simulink model "bcd_test"  (R2026a)
settings: Solver=ode15s
libraries: scuba_lib x3, nesl_utility x2, fl_lib x1
settings Model: DataDictionary=scubaParams.sldd  Creator=grouleau  LastModifiedBy=grouleau

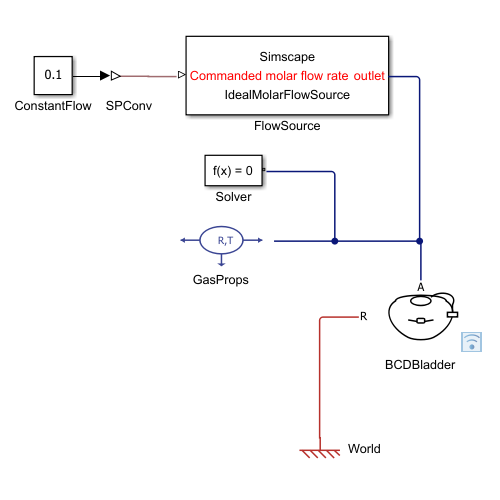
[thumbnail: Simulink's stored preview of the top-level diagram]
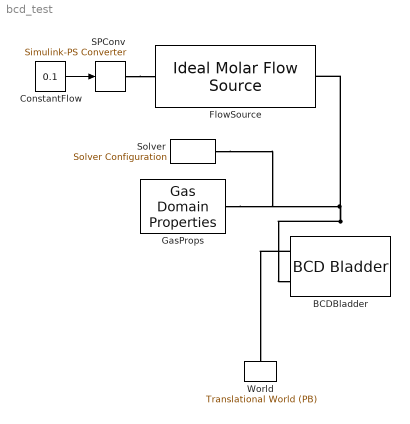
== system bcd_test ==
  BCDBladder : scuba_lib/gas/elements/BCD Bladder  V_max=0.015 m^3  n_init=0 mol  K_wall=1e7 Pa/m^3  rho_water=1025 kg/m^3  P_atm=101325 Pa  n_dot_in_specify=off  n_dot_in_priority=None  n_dot_in=0 mol/s  n_dot_in_nominal_specify=off  n_dot_in_nominal_value=1  n_dot_in_nominal_unit=mol/s  f_specify=off  f_priority=None  f=0 N  f_nominal_specify=off  f_nominal_value=1  f_nominal_unit=N  V_bcd_specify=off  V_bcd_priority=None  V_bcd=0 m^3  V_bcd_nominal_specify=off  V_bcd_nominal_value=1  V_bcd_nominal_unit=m^3
  ConstantFlow : Constant  Value=0.1
  FlowSource : scuba_lib/gas/elements/Ideal Molar Flow Source  n_dot_in_specify=off  n_dot_in_priority=None  n_dot_in=0 mol/s  n_dot_in_nominal_specify=off  n_dot_in_nominal_value=1  n_dot_in_nominal_unit=mol/s
  GasProps : scuba_lib/gas/elements/Gas Domain Properties  R_gas=8.314 J/(K*mol)  T=293.15 K  n_dot_thru_specify=off  n_dot_thru_priority=None  n_dot_thru=0 mol/s  n_dot_thru_nominal_specify=off  n_dot_thru_nominal_value=1  n_dot_thru_nominal_unit=mol/s
  SPConv : nesl_utility/Simulink-PS Converter  PhysicalDomain=network_engine_domain  SubClassName=ps_input  LeftPortType=input  RightPortType=output  PseudoPeriodic=off  Frequencies=[]  NoiseDistribution=none  NoiseParameters=[]  Unit=1  AffineConversion=off  FilteringAndDerivatives=provide  SimscapeFilterOrder=1  InputFilterTimeConstant=0.001  UdotUserProvided=0
  Solver : nesl_utility/Solver Configuration  PhysicalDomain=network_engine_domain  SubClassName=solver  LeftPortType=input  RightPortType=generic  Tones=[]  Harmonics=[]  SimulateNoise=off  Profile=off  UseLocalSampling=off  EnableSwitchedLinearOptims=on  FrequencyDomain=off  UseCCode=off  RelTol=0.001  AbsTol=0.001  MinStep=1e-09  ToWorkspace=off  RevertToSquareIcSolve=off  NumHomotopyIterations=100  PhasorMode=off  PhasorModeNumHarmonics=1  ConsistencySolver=NEWTON_XTOL_AFTER_FTOL  CanonicalOrdering=CANONICAL  OptimizeIntermediates=OPTIMIZED  IndexReductionMethod=DerivativeReplacement  DoDC=off  ResidualTolerance=1e-09  ConsistencyTolSource=GLOBAL  ConsistencyAbsTol=0.001  ConsistencyRelTol=0.001  ConsistencyTolFactor=0.001  UseLocalSolver=off  LocalSolverChoice=NE_BACKWARD_EULER_ADVANCER  ResolveIndetEquations=on  FunctionEvalNumThread=1  LocalSolverSampleTime=0.001  DoFixedCost=off  MaxNonlinIter=3  MaxModeIter=2  ComputeImpulses=off  ImpulseIterations=2  LinearAlgebra=auto  LinearAlgebraNumThread=0  EquationFormulation=NE_TIME_EF  DelaysMemoryBudget=1024  AutomaticFiltering=on  FilteringTimeConstant=0.001  PartitionStorageMethod=AS_NEEDED  PartitionMemoryBudget=1024  PartitionMethod=ROBUST  MultibodyUseLocalSolver=off  MultibodyLocalSolverChoice=ODE1  MultibodyLocalSolverSampleTime=0.001
  World : fl_lib/Translational/Elements/Translational World (PB)
  wires:
  ConstantFlow/1 -> SPConv/1
  connections:
  SPConv/RConn1 -- FlowSource/LConn1
  BCDBladder/LConn2 -- GasProps/LConn1 -- Solver/RConn1 -- FlowSource/RConn1
  BCDBladder/LConn1 -- World/RConn1
